simulink model "good_for_tabu"  (R2015a)
settings: Solver=ode45  StartTime=0.0  StopTime=10.0  RelTol=1e-3
values from neighbouring files (symbols this model uses):
  c = 5    [RD_Breach.m]    (also in RD_Breach_falsi.m; staliroHarness.m)
settings Model: Creator=jyotirmoy  LastModifiedBy=xjin
settings DebuggingCC: UnderspecifiedInitializationDetection=Classic  MergeDetectMultiDrivingBlocksExec=none  SolverPrmCheckMsg=warning

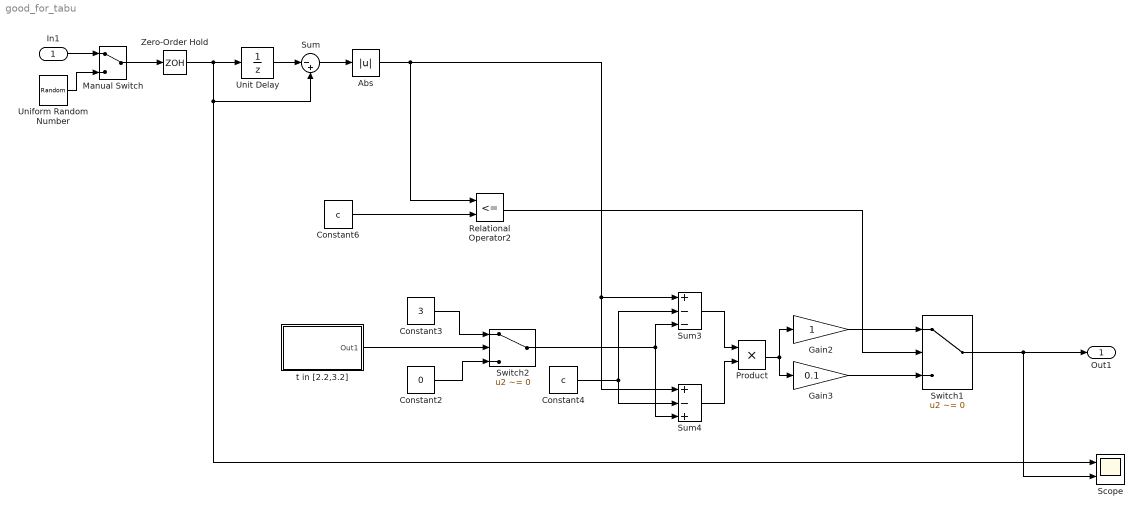
== system good_for_tabu ==
  In1 : Inport
  Abs : Abs
  Constant2 : Constant  Value=0
  Constant3 : Constant  Value=3
  Constant4 : Constant  Value=c
  Constant6 : Constant  Value=c
  Gain2 : Gain
  Gain3 : Gain  Gain=0.1
  Manual Switch : ManualSwitch
  Product : Product
  Relational Operator2 : RelationalOperator  Operator=<=  OutDataTypeStr=boolean
  Scope : Scope  NumInputPorts=2
      settings: TimeRange=10  YMin=-5~-5  YMax=5~5
  Sum : Sum  Inputs=|-+
  Sum3 : Sum  Inputs=+--
  Sum4 : Sum  Inputs=+-+
  Switch1 : Switch  Criteria=u2 ~= 0
  Switch2 : Switch  Criteria=u2 ~= 0
  Uniform Random Number : UniformRandomNumber  Minimum=0  Maximum=100  Seed=1  SampleTime=0.1
  Unit Delay : UnitDelay  InitialCondition=50  SampleTime=-1
  Zero-Order Hold : ZeroOrderHold  SampleTime=0.1
  t in [2.2,3.2] : Subsystem
  Out1 : Outport
  wires:
  Zero-Order Hold/1 -> Unit Delay/1, Sum/2, Scope/1
  Unit Delay/1 -> Sum/1
  Sum/1 -> Abs/1
  Abs/1 -> Sum4/1, Sum3/1, Relational Operator2/1
  In1/1 -> Manual Switch/1
  Manual Switch/1 -> Zero-Order Hold/1
  Uniform Random Number/1 -> Manual Switch/2
  Product/1 -> Gain3/1, Gain2/1
  Constant6/1 -> Relational Operator2/2
  Gain2/1 -> Switch1/1
  Gain3/1 -> Switch1/3
  Relational Operator2/1 -> Switch1/2
  t in [2.2,3.2]/1(Out1) -> Switch2/2
  Constant2/1 -> Switch2/3
  Constant3/1 -> Switch2/1
  Switch2/1 -> Sum3/3, Sum4/3
  Constant4/1 -> Sum4/2, Sum3/2
  Sum3/1 -> Product/1
  Sum4/1 -> Product/2
  Switch1/1 -> Scope/2, Out1/1

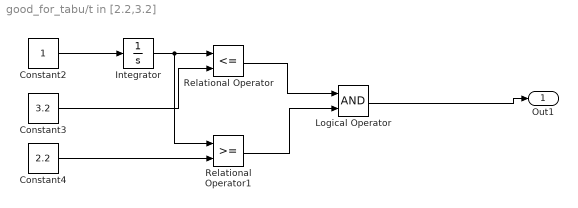
== system good_for_tabu/t in [2.2,3.2] ==
  Constant2 : Constant
  Constant3 : Constant  Value=3.2
  Constant4 : Constant  Value=2.2
  Integrator : Integrator
  Logical Operator : Logic  AllPortsSameDT=off  OutDataTypeStr=boolean
  Relational Operator : RelationalOperator  Operator=<=  OutDataTypeStr=boolean
  Relational Operator1 : RelationalOperator  OutDataTypeStr=boolean
  Out1 : Outport
  wires:
  Constant2/1 -> Integrator/1
  Integrator/1 -> Relational Operator/1, Relational Operator1/1
  Constant3/1 -> Relational Operator/2
  Constant4/1 -> Relational Operator1/2
  Relational Operator/1 -> Logical Operator/1
  Relational Operator1/1 -> Logical Operator/2
  Logical Operator/1 -> Out1/1
